simulink model "packetizer_test"  (Simulink 7.3)
settings: Solver=ode45  StartTime=0.0  StopTime=2000  RelTol=1e-3
libraries: xbsIndex_r4 x25
settings Model: Creator=tfiliba  LastModifiedBy=tfiliba

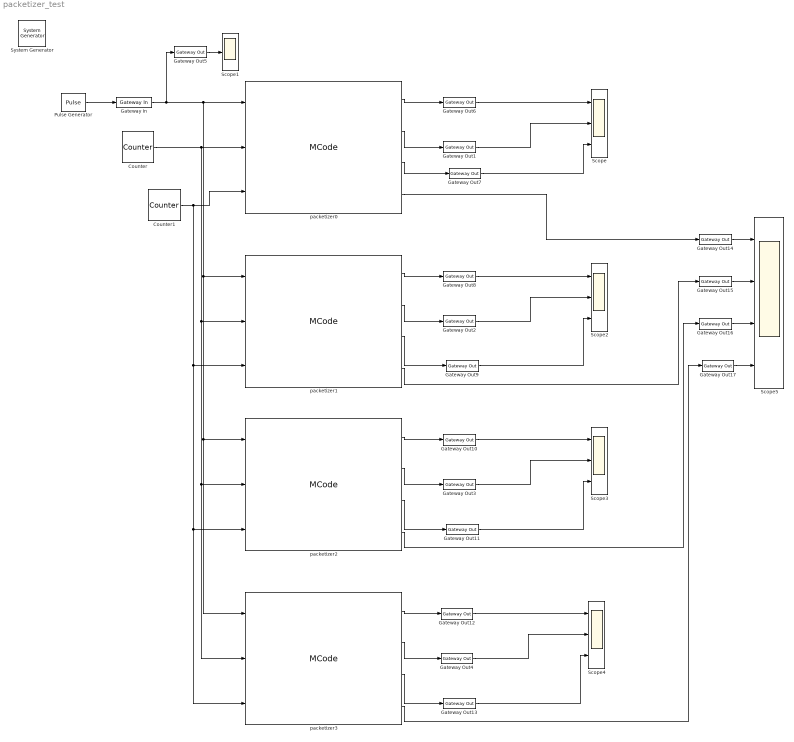
== system packetizer_test ==
  " System Generator" : xbsIndex_r4/ System Generator  Tag=genX  SystemSampleTime=-1  xilinxfamily=Virtex6  part=xc6vsx315t  speed=-3  package=ff1156  synthesis_tool=XST  clock_wrapper=Clock Enables  directory=./netlist  testbench=off  simulink_period=1  sysclk_period=10  dcm_input_clock_period=10  incr_netlist=off  trim_vbits=Everywhere in SubSystem  dbl_ovrd=According to Block Masks  core_generation=According to Block Masks  run_coregen=off  deprecated_control=off  eval_field=0  block_type=sysgen
      settings: block_version=11.4
  Counter : xbsIndex_r4/Counter  cnt_type=Count Limited  cnt_to=5  operation=Up  start_count=0  cnt_by_val=1  arith_type=Unsigned  n_bits=64  bin_pt=0  load_pin=off  rst=off  en=off  explicit_period=on  period=1  dbl_ovrd=off  use_behavioral_HDL=off  implementation=Fabric  block_type=counter
      settings: block_version=11.4
  Counter1 : xbsIndex_r4/Counter  cnt_type=Count Limited  cnt_to=1  operation=Up  start_count=0  cnt_by_val=1  arith_type=Unsigned  n_bits=64  bin_pt=0  load_pin=off  rst=off  en=off  explicit_period=on  period=1  dbl_ovrd=off  use_behavioral_HDL=off  implementation=Fabric  block_type=counter
      settings: block_version=11.4
  Gateway In : xbsIndex_r4/Gateway In  arith_type=Boolean  n_bits=16  bin_pt=14  quantization="Round  (unbiased: +/- Inf)"  overflow=Saturate  period=1  dbl_ovrd=off  timing_constraint=None  locs_specified=off  LOCs={}  hdl_port=on  block_type=gatewayin
      settings: infoedit="Gateway in block.  Converts inputs of type Simulink integer, double and fixed point to  Xilinx fixed point type.<br><br>Hardware notes:  In hardware these blocks become top level input ports."  block_version=11.4
  Gateway Out{1..17} (17 alike) : xbsIndex_r4/Gateway Out  hdl_port=off  timing_constraint=None  locs_specified=off  LOCs={}  block_type=gatewayout
      settings: infoedit="Gateway out block.  Converts Xilinx fixed point inputs into ouputs of type Simulink integer, double, or fixed point.<br><br>Hardware notes:  In hardware these blocks become top level output ports or are discarded, depending on how they are configured."  block_version=11.4
  Pulse Generator : DiscretePulseGenerator  Amplitude=1  Period=256  PulseWidth=1  PhaseDelay=5  SampleTime=1
  Scope{,2..4} (4 alike) : Scope  NumInputPorts=3
      Scope settings: YMin=-5~-5~-5  YMax=5~5~5
      Scope2 settings: YMin=-5~-5~-5  YMax=5~5~5  SaveName=ScopeData2
      Scope3 settings: YMin=-5~-5~-5  YMax=5~5~5  SaveName=ScopeData3
      Scope4 settings: YMin=-5~-5~-5  YMax=5~5~5  SaveName=ScopeData4
  Scope1 : Scope
  Scope5 : Scope  NumInputPorts=4
      settings: YMin=-5~-5~-5~-5  YMax=5~5~5~5  SaveName=ScopeData5
  packetizer0 : xbsIndex_r4/MCode  mfname=packetizer  explicit_period=off  period=1  inputsTable={'boundInpExpr'=>['','','','16','16','4','0'],'inputs'=>['sync','din','sys_counter','packet_size','numcomputers','numtengbe','tengbe_id']}  outputsTable={'outputs'=>['dout','valid','end_of_frame','st'],'suppressOut'=>['off','off','off','on']}  dbl_ovrd=off  enable_stdout=off  enable_debug=off  suppress_output=on  defparams={'packet_size',16,'numcomputers',16,'numtengbe',4,'tengbe_id',0}  hide_port_list={'st'}  block_type=mcode
      settings: block_version=11.4
  packetizer1 : xbsIndex_r4/MCode  mfname=packetizer  explicit_period=off  period=1  inputsTable={'boundInpExpr'=>['','','','16','16','4','1'],'inputs'=>['sync','din','sys_counter','packet_size','numcomputers','numtengbe','tengbe_id']}  outputsTable={'outputs'=>['dout','valid','end_of_frame','st'],'suppressOut'=>['off','off','off','on']}  dbl_ovrd=off  enable_stdout=off  enable_debug=off  suppress_output=on  defparams={'packet_size',16,'numcomputers',16,'numtengbe',4,'tengbe_id',1}  hide_port_list={'st'}  block_type=mcode
      settings: block_version=11.4
  packetizer2 : xbsIndex_r4/MCode  mfname=packetizer  explicit_period=off  period=1  inputsTable={'boundInpExpr'=>['','','','16','16','4','2'],'inputs'=>['sync','din','sys_counter','packet_size','numcomputers','numtengbe','tengbe_id']}  outputsTable={'outputs'=>['dout','valid','end_of_frame','st'],'suppressOut'=>['off','off','off','on']}  dbl_ovrd=off  enable_stdout=off  enable_debug=off  suppress_output=on  defparams={'packet_size',16,'numcomputers',16,'numtengbe',4,'tengbe_id',2}  hide_port_list={'st'}  block_type=mcode
      settings: block_version=11.4
  packetizer3 : xbsIndex_r4/MCode  mfname=packetizer  explicit_period=off  period=1  inputsTable={'boundInpExpr'=>['','','','16','16','4','3'],'inputs'=>['sync','din','sys_counter','packet_size','numcomputers','numtengbe','tengbe_id']}  outputsTable={'outputs'=>['dout','valid','end_of_frame','st'],'suppressOut'=>['off','off','off','on']}  dbl_ovrd=off  enable_stdout=off  enable_debug=off  suppress_output=on  defparams={'packet_size',16,'numcomputers',16,'numtengbe',4,'tengbe_id',3}  hide_port_list={'st'}  block_type=mcode
      settings: block_version=11.4
  wires:
  Gateway In/1 -> packetizer1/1, packetizer2/1, packetizer3/1, packetizer0/1, Gateway Out5/1
  Counter/1 -> packetizer0/2, packetizer1/2, packetizer2/2, packetizer3/2
  Counter1/1 -> packetizer0/3, packetizer1/3, packetizer2/3, packetizer3/3
  packetizer0/2 -> Gateway Out1/1
  Pulse Generator/1 -> Gateway In/1
  Gateway Out5/1 -> Scope1/1
  packetizer0/1 -> Gateway Out6/1
  packetizer0/3 -> Gateway Out7/1
  Gateway Out6/1 -> Scope/1
  Gateway Out1/1 -> Scope/2
  Gateway Out7/1 -> Scope/3
  packetizer1/2 -> Gateway Out2/1
  packetizer1/1 -> Gateway Out8/1
  packetizer1/3 -> Gateway Out9/1
  Gateway Out8/1 -> Scope2/1
  Gateway Out2/1 -> Scope2/2
  Gateway Out9/1 -> Scope2/3
  packetizer2/2 -> Gateway Out3/1
  packetizer2/1 -> Gateway Out10/1
  packetizer2/3 -> Gateway Out11/1
  Gateway Out10/1 -> Scope3/1
  Gateway Out3/1 -> Scope3/2
  Gateway Out11/1 -> Scope3/3
  packetizer3/2 -> Gateway Out4/1
  packetizer3/1 -> Gateway Out12/1
  packetizer3/3 -> Gateway Out13/1
  Gateway Out12/1 -> Scope4/1
  Gateway Out4/1 -> Scope4/2
  Gateway Out13/1 -> Scope4/3
  packetizer3/4 -> Gateway Out17/1
  Gateway Out17/1 -> Scope5/4
  packetizer2/4 -> Gateway Out16/1
  packetizer1/4 -> Gateway Out15/1
  Gateway Out15/1 -> Scope5/2
  Gateway Out16/1 -> Scope5/3
  Gateway Out14/1 -> Scope5/1
  packetizer0/4 -> Gateway Out14/1
